simulink model "SequenceSeparation"  (R2018a)
settings: Solver=ode5  StartTime=0.0  StopTime=1  FixedStep=Ts  RelTol=1e-3
values from neighbouring files (symbols this model uses):
  Cdc = 2 * Sn * H / Vdc^2    (= 0.01875)    [SequenceSeparation_script.m]
  Cf = 1 / (wn * Xf)    (= 0.000159154943092)    [SequenceSeparation_script.m]
  Fn = 50    [SequenceSeparation_script.m]
  Kp_current = Rr * (Ti_current - halfTs)/(Tsum + halfTs)    [SequenceSeparation_script.m]
  Lr = Vdc / (0.8 * 2^0.5 * ( Sn / 3^0.5 / Vrms) * Fsw)    (= 0.00075)    [SequenceSeparation_script.m]
  Rf = 1 / ( 3 * 2 * pi * fres * Cf)    [SequenceSeparation_script.m]
  Rr = 0.005    [SequenceSeparation_script.m]
  Rt = 0.005    [SequenceSeparation_script.m]
  Sn = 1.5    [SequenceSeparation_script.m]
  Ts = 1e-6    (= 1e-06)    [SequenceSeparation_script.m]
  Ts_cont = 1/10000    (= 0.0001)    [SequenceSeparation_script.m]
  Ts_pwm = 1/200000    (= 5e-06)    [SequenceSeparation_script.m]
  Vdc = 2    [SequenceSeparation_script.m]
  Vrms = (3/2)^0.5    (= 1.22474487139)    [SequenceSeparation_script.m]
  Xr = Lr * wn    (= 0.235619449019)    [SequenceSeparation_script.m]
  Xt = 0.08    [SequenceSeparation_script.m]
undefined symbols (not defined in the file or in its folder): D1, Delta
libraries: powerlib x30, pwrsysVICtrl_202301 x6, pwrsysVSrc_202301 x2, pwrsysBasic_202301 x2, powerlib_meascontrol x1, pwrsysTransf_202301 x1
settings Model: Creator=daniemot  LastModifiedBy=daniemot

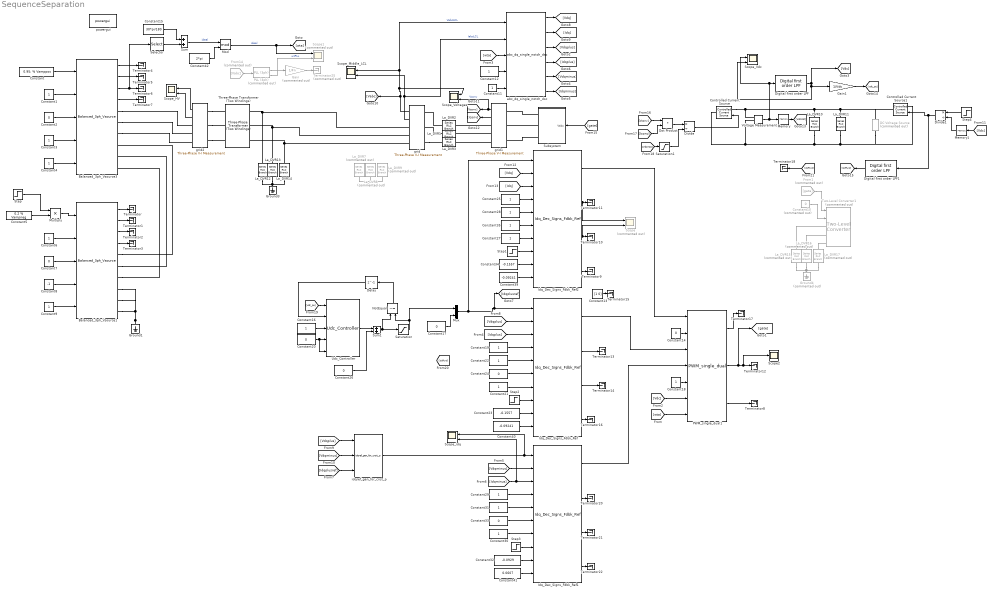
== system SequenceSeparation ==
  Balanced_3ph_Vsource1 : pwrsysVSrc_202301/Balanced_3ph_Vsource  BaseAmp=1  fn=50  AmpIni=1  SeqIni=1  AngIni=0  FIni=50  HarmIni=1
  Balanced_3ph_Vsource3 : pwrsysVSrc_202301/Balanced_3ph_Vsource  BaseAmp=1  fn=50  AmpIni=1  SeqIni=1  AngIni=0  FIni=50  HarmIni=1
  Constant : Constant  Value=0.95; % Vamppos
  Constant{1,3..4,6,9,11..12,16,18..19,21..22,25,27..31,35} (19 alike) : Constant
  Constant10 : Constant  Commented=on  Value=0
  Constant13 : Constant  Value=[1 0]
  Constant{2,7,14,17,20,24,26,33} (8 alike) : Constant  Value=0
  Constant15 : Constant  Value=30*pi/180
  Constant23 : Constant  Value=-0.1557
  Constant32 : Constant  Value=-0.0929
  Constant34 : Constant  Value=-0.1557
  Constant39 : Constant  Value=-0.09241
  Constant40 : Constant  Value=-0.09241
  Constant41 : Constant  Value=0.0607
  Constant42 : Constant  Value=2*pi
  Constant5 : Constant  Value=0.2 % Vampneg
  Constant8 : Constant  Value=-1
  Controlled Current Source : powerlib/Electrical Sources/Controlled Current Source  Initialize=on  Source_Type=AC  Amplitude=0  Phase=0  Frequency=0  Measurements=None
  Controlled Current Source1 : powerlib/Electrical Sources/Controlled Current Source  Initialize=on  Source_Type=AC  Amplitude=0  Phase=0  Frequency=0  Measurements=None
  DC Voltage Source : powerlib/Electrical Sources/DC Voltage Source  Commented=on  Amplitude=Vdc  Measurements=None
  Delay : Delay  DelayLength=1  SampleTime=Ts_cont
  Digital first order LPF : pwrsysBasic_202301/Digital first order LPF  Ts=Ts_cont  fcutout=fres
  Digital first order LPF1 : pwrsysBasic_202301/Digital first order LPF  Ts=Ts_cont  fcutout=fres
  Divide : Product  Inputs=*/
  Divide1 : Product  Inputs=*/
  Dot Product : DotProduct  InputSameDT=on  OutDataTypeStr=Inherit: Inherit via internal rule
  From1 : From  Commented=on  GotoTag=gate
  From14 : From  Commented=on  GotoTag=Vabc
  Gain : Gain  Commented=on  Gain=1/Fn
  Gain1 : Gain  Gain=1/Vdc
  Ground1 : powerlib/Elements/Ground  LConnTagsString=a
  Ground3 : powerlib/Elements/Ground  LConnTagsString=a
  Ground4 : powerlib/Elements/Ground  Commented=on  LConnTagsString=a
  Idq_Dec_Signs_Fdbk_Ref : pwrsysVICtrl_202301/Idq_Dec_Signs_Fdbk_Ref  Ts=Ts_cont  fn=Fn  Kp=Kp_current  Ti=Ti_current  L=Xr  PI_max=1.5  PI_min=-1.5  TrafoPhaseComp=0
  Idq_Dec_Signs_Fdbk_Ref1 : pwrsysVICtrl_202301/Idq_Dec_Signs_Fdbk_Ref  Ts=Ts_cont  fn=Fn  Kp=Kp_current  Ti=Ti_current  L=Xr  PI_max=1.5  PI_min=-1.5  TrafoPhaseComp=0
  Idq_Dec_Signs_Fdbk_Ref2 : pwrsysVICtrl_202301/Idq_Dec_Signs_Fdbk_Ref  Ts=Ts_cont  fn=Fn  Kp=Kp_current  Ti=Ti_current  L=Xr  PI_max=1.5  PI_min=-1.5  TrafoPhaseComp=0
  La_DVR1 : powerlib/Elements/Series RLC Branch  LConnTagsString=__new0  RConnTagsString=__new0  BranchType=RL  Resistance=Rr  Inductance=Lr  SetiL0=off  InitialCurrent=0  Capacitance=1.0  Setx0=off  InitialVoltage=0  Measurements=None
  La_DVR10 : powerlib/Elements/Series RLC Branch  LConnTagsString=__new0  RConnTagsString=__new0  BranchType=R  Resistance=100000  Inductance=0.3/(2*pi*50)  SetiL0=off  InitialCurrent=0  Capacitance=Cf  Setx0=off  InitialVoltage=0  Measurements=None
  La_DVR11 : powerlib/Elements/Series RLC Branch  LConnTagsString=__new0  RConnTagsString=__new0  BranchType=C  Resistance=100000  Inductance=0.3/(2*pi*50)  SetiL0=off  InitialCurrent=0  Capacitance=Cdc  Setx0=on  InitialVoltage=Vdc  Measurements=None
  La_DVR12 : powerlib/Elements/Series RLC Branch  LConnTagsString=__new0  RConnTagsString=__new0  BranchType=R  Resistance=1e6  Inductance=0.3/(2*pi*50)  SetiL0=off  InitialCurrent=0  Capacitance=1.0  Setx0=off  InitialVoltage=0  Measurements=None
  La_DVR13 : powerlib/Elements/Series RLC Branch  LConnTagsString=__new0  RConnTagsString=__new0  BranchType=R  Resistance=1e6  Inductance=0.3/(2*pi*50)  SetiL0=off  InitialCurrent=0  Capacitance=1.0  Setx0=off  InitialVoltage=0  Measurements=None
  La_DVR14 : powerlib/Elements/Series RLC Branch  LConnTagsString=__new0  RConnTagsString=__new0  BranchType=R  Resistance=1e6  Inductance=0.3/(2*pi*50)  SetiL0=off  InitialCurrent=0  Capacitance=1.0  Setx0=off  InitialVoltage=0  Measurements=None
  La_DVR15 : powerlib/Elements/Series RLC Branch  Commented=on  LConnTagsString=__new0  RConnTagsString=__new0  BranchType=R  Resistance=1e6  Inductance=0.3/(2*pi*50)  SetiL0=off  InitialCurrent=0  Capacitance=1.0  Setx0=off  InitialVoltage=0  Measurements=None
  La_DVR16 : powerlib/Elements/Series RLC Branch  Commented=on  LConnTagsString=__new0  RConnTagsString=__new0  BranchType=R  Resistance=1e6  Inductance=0.3/(2*pi*50)  SetiL0=off  InitialCurrent=0  Capacitance=1.0  Setx0=off  InitialVoltage=0  Measurements=None
  La_DVR17 : powerlib/Elements/Series RLC Branch  Commented=on  LConnTagsString=__new0  RConnTagsString=__new0  BranchType=R  Resistance=1e6  Inductance=0.3/(2*pi*50)  SetiL0=off  InitialCurrent=0  Capacitance=1.0  Setx0=off  InitialVoltage=0  Measurements=None
  La_DVR2 : powerlib/Elements/Series RLC Branch  LConnTagsString=__new0  RConnTagsString=__new0  BranchType=RL  Resistance=Rr  Inductance=Lr  SetiL0=off  InitialCurrent=0  Capacitance=1.0  Setx0=off  InitialVoltage=0  Measurements=None
  La_DVR3 : powerlib/Elements/Series RLC Branch  LConnTagsString=__new0  RConnTagsString=__new0  BranchType=RL  Resistance=Rr  Inductance=Lr  SetiL0=off  InitialCurrent=0  Capacitance=1.0  Setx0=off  InitialVoltage=0  Measurements=None
  La_DVR7 : powerlib/Elements/Series RLC Branch  Commented=on  LConnTagsString=__new0  RConnTagsString=__new0  BranchType=RC  Resistance=Rf  Inductance=0.3/(2*pi*50)  SetiL0=off  InitialCurrent=0  Capacitance=Cf  Setx0=off  InitialVoltage=0  Measurements=None
  La_DVR8 : powerlib/Elements/Series RLC Branch  Commented=on  LConnTagsString=__new0  RConnTagsString=__new0  BranchType=RC  Resistance=Rf  Inductance=0.3/(2*pi*50)  SetiL0=off  InitialCurrent=0  Capacitance=Cf  Setx0=off  InitialVoltage=0  Measurements=None
  La_DVR9 : powerlib/Elements/Series RLC Branch  Commented=on  LConnTagsString=__new0  RConnTagsString=__new0  BranchType=RC  Resistance=Rf  Inductance=0.3/(2*pi*50)  SetiL0=off  InitialCurrent=0  Capacitance=Cf  Setx0=off  InitialVoltage=0  Measurements=None
  Memory : Memory
  Memory1 : Memory  InitialCondition=1
  Mod : Math  Operator=mod  SaturateOnIntegerOverflow=on
  Multiply : Product
  Mux : Mux  Inputs=2
  NotEqual : RelationalOperator  Operator=~=  OutDataTypeStr=boolean  RndMeth=Simplest
  PLL (3ph) : powerlib_meascontrol/PLL/PLL (3ph)  Commented=on  Fmin=0.8*Fn  Par_Init=[0, Fn]  ParK=[180, 3200, 1]  TcD=1e-4  MaxRateChangeFreq=12  FilterCutOffFreq=25  Ts=Ts_cont  AGC=on
  PWM_single_dual1 : pwrsysVICtrl_202301/PWM_single_dual  fsw=Fsw  Ts=Ts_pwm  Uabp=Vampline  PWM_Ini_Phase=90
  Saturation : Saturate  UpperLimit=1.5  LowerLimit=-1.5
  Saturation1 : Saturate  UpperLimit=5  LowerLimit=0.25
  Scope : Scope  Commented=on  NumInputPorts=2
  Scope1 : Scope  Commented=on  NumInputPorts=2
  Scope2 : Scope
  Scope_HV : Scope  NumInputPorts=2
  Scope_Middle_LCL : Scope  NumInputPorts=2
  "Scope_Vdc " : Scope  NumInputPorts=2
  Scope_Voltages : Scope  NumInputPorts=2
  Scope_idq : Scope  NumInputPorts=2
  Selector : Selector  InputPortWidth=3  IndexOptions=Index vector (dialog)  Indices=[1]  OutputSizes=1
  Step : Step  Time=0.5  SampleTime=0
  Step1 : Step  Time=0.0002  After=0  SampleTime=0
  Step2 : Step  Time=0.0002  After=0  SampleTime=0
  Step3 : Step  Time=0.0002  After=0  SampleTime=0
  Step4 : Step  Time=0.25  After=0.25  SampleTime=0
  Subsystem : Subsystem
  Sum : Sum
  Sum1 : Sum
  Terminator{,1..18,20..22} (22 alike) : Terminator
  Terminator25 : Terminator  Commented=on
  Three-Phase Transformer (Two Windings) : powerlib/Elements/Three-Phase Transformer (Two Windings)  Winding1Connection=Delta (D1)  Winding2Connection=Y  CoreType=Three single-phase transformers  SetSaturation=off  Hysteresis=off  DataFile='hysteresis'  SetInitialFlux=off  Measurements=None  UNITS=pu  NominalPower=[ Sn , Fn ]  Winding1=[ Vrms , Rt , Xt ]  Winding2=[ Vrms , Rt , Xt ]  Rm=500  Lm=500  L0=0.5  Saturation=[ 0,0 ; 0.0024,1.2 ; 1.0,1.52 ]  InitialFluxes=[ 0.8 , -0.8 , 0.7 ]  MoreParameters=off  BreakLoop=off  DataType=off  TransfoNumber=1
  Two-Level Converter1 : powerlib/Power Electronics/Two-Level Converter  Commented=on  ModelType=Average model (Uref-controlled)  Ron=0.00001  Rs=1e6  Cs=inf  Vforward=[0,0]  Ron_Diode=0.001e-3  Rs_Diode=1e6  Cs_Diode=inf  Vf_Diode=1e-6  Rs_CurrentSource=inf
      settings: SourceProductName=Simscape Power Systems  SourceProductBaseCode=PS
  Udc_Controller : pwrsysVICtrl_202301/Udc_Controller  Ts=Ts_cont  Kp=5  Ti=0.025  PI_max=1.5  PI_min=-1.5
  Voltage Measurement : powerlib/Measurements/Voltage Measurement  PhasorSimulation=off  OutputType=Complex  PSBequivalent=0
  abc_dq_single_notch_dsc : pwrsysTransf_202301/abc_dq_single_notch_dsc  Ts=Ts_cont  fn=2*Fn  zeta=0.707
  grid : powerlib/Measurements/Three-Phase V-I Measurement  VoltageMeasurement=phase-to-ground  SetLabelV=off  LabelV=vgrid  Vpu=off  VpuLL=off  CurrentMeasurement=yes  SetLabelI=off  LabelI=igrid  Ipu=off  Pbase=sn  Vbase=uab  OutputType=Complex  PhasorSimulation=off  PSBequivalent=0
  grid1 : powerlib/Measurements/Three-Phase V-I Measurement  VoltageMeasurement=phase-to-ground  SetLabelV=off  LabelV=vgrid  Vpu=off  VpuLL=off  CurrentMeasurement=yes  SetLabelI=off  LabelI=igrid  Ipu=off  Pbase=sn  Vbase=uab  OutputType=Complex  PhasorSimulation=off  PSBequivalent=0
  grid2 : powerlib/Measurements/Three-Phase V-I Measurement  VoltageMeasurement=phase-to-ground  SetLabelV=off  LabelV=vgrid  Vpu=off  VpuLL=off  CurrentMeasurement=yes  SetLabelI=off  LabelI=igrid  Ipu=off  Pbase=sn  Vbase=uab  OutputType=Complex  PhasorSimulation=off  PSBequivalent=0
  idqref_gen_for_cnst_p : pwrsysVICtrl_202301/idqref_gen_for_cnst_p  Ts_control=Ts_cont
  powergui : powerlib/powergui  Priority=1  SimulationMode=Discrete  SampleTime=Ts  frequency=60  Iterations=50  frequencyindice=0  Pbase=100e6  ErrMax=1e-4  UnitsV=kV  UnitsW=MW  buscounter=0  FunctionMessages=off  echomessages=off  EnableUseOfTLC=off  CurrentSourceSwitches=off  DisableSnubberDevices=off  DisableRonSwitches=off  DisableVfSwitches=off  DisplayEquations=off  SolverType=Tustin/Backward Euler (TBE)  Interpol=off  ExternalGateDelay=off  methode=off  Ts=100  x0status=blocks  SPID=off  SwTol=0  HookPort=off  RestoreLinks=warning  ResistiveCurrentMeasurement=off  Frange=[60:1:1600]  Ylog=on  Xlog=on  ShowGrid=on  save=off  variable=ZData  structure=0  ZoomFFT=off  StartTime=0.0  cycles=1  DisplayStyle=1  fundamental=60  FreqAxis=off  MaxFrequency=1000  frequencyindicesteady=1  RmsSteady=1  display=off
  wires:
  Constant/1 -> Balanced_3ph_Vsource3/1
  Constant1/1 -> Balanced_3ph_Vsource3/2
  Constant2/1 -> Balanced_3ph_Vsource3/3
  Constant3/1 -> Balanced_3ph_Vsource3/4
  Constant4/1 -> Balanced_3ph_Vsource3/5
  Constant8/1 -> Balanced_3ph_Vsource1/4
  Constant5/1 -> Multiply/2
  Constant9/1 -> Balanced_3ph_Vsource1/5
  Constant6/1 -> Balanced_3ph_Vsource1/2
  Constant7/1 -> Balanced_3ph_Vsource1/3
  Balanced_3ph_Vsource1/1 -> Terminator/1
  Balanced_3ph_Vsource1/2 -> Terminator1/1
  Balanced_3ph_Vsource1/3 -> Terminator2/1
  Balanced_3ph_Vsource1/4 -> Terminator3/1
  Balanced_3ph_Vsource3/1 -> Terminator4/1
  Balanced_3ph_Vsource3/4 -> Terminator7/1
  Balanced_3ph_Vsource3/2 -> Terminator5/1
  Balanced_3ph_Vsource3/3 -> Selector/1, Terminator6/1
  Selector/1 -> Sum/2
  Mod/1 -> Scope1/1, [wta]  "ideal"
  Constant15/1 -> Sum/1
  Saturation/1 -> Mux/1, NotEqual/2
  [wta] -> PWM_single_dual1/7
  Constant10/1 -> Two-Level Converter1/2
  From1/1 -> Two-Level Converter1/1
  PWM_single_dual1/2 -> [gate], Scope2/1, Terminator12/1
  Constant11/1 -> abc_dq_single_notch_dsc/5
  [wta] -> abc_dq_single_notch_dsc/3
  Constant12/1 -> abc_dq_single_notch_dsc/4
  [Vdc] -> PWM_single_dual1/6
  PWM_single_dual1/1 -> Terminator17/1
  PWM_single_dual1/3 -> Terminator8/1
  Constant14/1 -> PWM_single_dual1/2
  Constant18/1 -> PWM_single_dual1/5
  Constant19/1 -> Idq_Dec_Signs_Fdbk_Ref/4
  Constant21/1 -> Idq_Dec_Signs_Fdbk_Ref/7
  Constant22/1 -> Idq_Dec_Signs_Fdbk_Ref/5
  Constant24/1 -> Idq_Dec_Signs_Fdbk_Ref/6
  [Vdqplus] -> Idq_Dec_Signs_Fdbk_Ref/2
  Idq_Dec_Signs_Fdbk_Ref/2 -> Terminator13/1
  Idq_Dec_Signs_Fdbk_Ref/3 -> Terminator14/1
  Idq_Dec_Signs_Fdbk_Ref/4 -> Terminator16/1
  grid/1 -> [Vabc], Scope_Voltages/1, abc_dq_single_notch_dsc/1, Scope_Middle_LCL/1  "VabcLCL"
  grid/2 -> abc_dq_single_notch_dsc/2, Scope_Middle_LCL/2  "IabcLCL"
  grid1/1 -> [Vconv], Scope_Voltages/2  "Vconv"
  grid1/2 -> [Iconv]
  Multiply/1 -> Balanced_3ph_Vsource1/1
  Step/1 -> Multiply/1
  Constant29/1 -> Idq_Dec_Signs_Fdbk_Ref1/4
  [Vdqminus] -> Idq_Dec_Signs_Fdbk_Ref1/2
  Idq_Dec_Signs_Fdbk_Ref1/2 -> Terminator20/1
  [Idqminus] -> Scope_idq/2, Idq_Dec_Signs_Fdbk_Ref1/3
  Idq_Dec_Signs_Fdbk_Ref1/3 -> Terminator21/1
  Constant30/1 -> Idq_Dec_Signs_Fdbk_Ref1/7
  Idq_Dec_Signs_Fdbk_Ref1/4 -> Terminator22/1
  Constant33/1 -> Idq_Dec_Signs_Fdbk_Ref1/6
  Constant31/1 -> Idq_Dec_Signs_Fdbk_Ref1/5
  abc_dq_single_notch_dsc/3 -> [Vdqplus]
  abc_dq_single_notch_dsc/5 -> [Vdqminus]
  abc_dq_single_notch_dsc/6 -> [Idqminus]
  abc_dq_single_notch_dsc/4 -> [Idqplus]
  [Idqplusref] -> idqref_gen_for_cnst_p/3
  [Vdqplus] -> idqref_gen_for_cnst_p/1
  [Vdqminus] -> idqref_gen_for_cnst_p/2
  abc_dq_single_notch_dsc/1 -> [Vdq]
  abc_dq_single_notch_dsc/2 -> [Idq]
  Constant20/1 -> Udc_Controller/5, Udc_Controller/4
  Constant16/1 -> Udc_Controller/3
  Udc_Controller/1 -> Sum1/1
  Sum1/1 -> NotEqual/1, Saturation/1
  Constant26/1 -> Sum1/2
  Delay/1 -> Udc_Controller/2
  Digital first order LPF/1 -> Gain1/1, "Scope_Vdc "/2, [Vdc]
  Voltage Measurement/1 -> Memory/1, Digital first order LPF/1, "Scope_Vdc "/1
  [vdc_pu] -> Udc_Controller/1
  Constant25/1 -> Idq_Dec_Signs_Fdbk_Ref2/4
  Constant28/1 -> Idq_Dec_Signs_Fdbk_Ref2/5
  Constant35/1 -> Idq_Dec_Signs_Fdbk_Ref2/6
  Constant27/1 -> Idq_Dec_Signs_Fdbk_Ref2/7
  Step1/1 -> Idq_Dec_Signs_Fdbk_Ref2/8
  [Vdq] -> Idq_Dec_Signs_Fdbk_Ref2/2
  [Idq] -> Idq_Dec_Signs_Fdbk_Ref2/3
  Idq_Dec_Signs_Fdbk_Ref2/4 -> Terminator9/1
  Idq_Dec_Signs_Fdbk_Ref2/3 -> Scope/2, Terminator10/1
  Idq_Dec_Signs_Fdbk_Ref2/2 -> Scope/1, Terminator11/1
  Constant13/1 -> Terminator15/1
  Idq_Dec_Signs_Fdbk_Ref2/1 -> PWM_single_dual1/1
  idqref_gen_for_cnst_p/1 -> Scope_idq/1, Idq_Dec_Signs_Fdbk_Ref1/1
  grid2/1 -> Scope_HV/1
  grid2/2 -> Scope_HV/2
  Constant34/1 -> Idq_Dec_Signs_Fdbk_Ref2/9
  Constant39/1 -> Idq_Dec_Signs_Fdbk_Ref2/10
  Step2/1 -> Idq_Dec_Signs_Fdbk_Ref/8
  Constant40/1 -> Idq_Dec_Signs_Fdbk_Ref/10
  Constant23/1 -> Idq_Dec_Signs_Fdbk_Ref/9
  Constant32/1 -> Idq_Dec_Signs_Fdbk_Ref1/9
  Constant41/1 -> Idq_Dec_Signs_Fdbk_Ref1/10
  Step3/1 -> Idq_Dec_Signs_Fdbk_Ref1/8
  From14/1 -> PLL (3ph)/1
  PLL (3ph)/1 -> Gain/1
  Gain/1 -> Terminator25/1
  PLL (3ph)/2 -> Scope1/2  "wtPLL"
  Sum/1 -> Mod/1  "ideal"
  Constant42/1 -> Mod/2
  [Idqplus] -> Idq_Dec_Signs_Fdbk_Ref/3
  Idq_Dec_Signs_Fdbk_Ref/1 -> PWM_single_dual1/3
  Idq_Dec_Signs_Fdbk_Ref1/1 -> PWM_single_dual1/4
  [gate] -> Subsystem/1(Vabc)
  [Vconv] -> Dot Product/1
  [Iconv] -> Dot Product/2
  Memory/1 -> [Vdcinst]
  Dot Product/1 -> Divide/1
  [Vdcinst] -> Saturation1/1
  Saturation1/1 -> Divide/2
  Divide/1 -> Controlled Current Source/1
  NotEqual/1 -> Delay/1
  Gain1/1 -> [vdc_pu]
  Mux/1 -> Idq_Dec_Signs_Fdbk_Ref2/1, [Idqplusref], Idq_Dec_Signs_Fdbk_Ref/1
  Constant17/1 -> Mux/2
  Step4/1 -> Divide1/1
  Divide1/1 -> Digital first order LPF1/1, Controlled Current Source1/1
  [Vdc] -> Memory1/1
  Memory1/1 -> Divide1/2
  Digital first order LPF1/1 -> [idcffwrd]
  [idcffwrd] -> Terminator18/1
  connections:
  Ground1/LConn1 -- Balanced_3ph_Vsource1/RConn6 -- Balanced_3ph_Vsource1/RConn5 -- Balanced_3ph_Vsource1/RConn4
  Balanced_3ph_Vsource1/RConn3 -- Balanced_3ph_Vsource3/RConn6
  Balanced_3ph_Vsource1/RConn2 -- Balanced_3ph_Vsource3/RConn5
  Balanced_3ph_Vsource1/RConn1 -- Balanced_3ph_Vsource3/RConn4
  Balanced_3ph_Vsource3/RConn1 -- grid2/RConn1
  Balanced_3ph_Vsource3/RConn2 -- grid2/RConn2
  Balanced_3ph_Vsource3/RConn3 -- grid2/RConn3
  Voltage Measurement/LConn1 -- DC Voltage Source/RConn1 -- Controlled Current Source1/RConn1 -- La_DVR11/LConn1 -- La_DVR10/LConn1 -- Controlled Current Source/LConn1
  Voltage Measurement/LConn2 -- Controlled Current Source/RConn1 -- DC Voltage Source/LConn1 -- Controlled Current Source1/LConn1 -- La_DVR11/RConn1 -- La_DVR10/RConn1
  La_DVR9/LConn1 -- La_DVR7/LConn1 -- La_DVR8/LConn1
  grid1/RConn1 -- La_DVR2/LConn1
  grid1/RConn2 -- La_DVR1/LConn1
  grid1/RConn3 -- La_DVR3/LConn1
  grid/LConn3 -- La_DVR3/RConn1
  La_DVR1/RConn1 -- grid/LConn2
  La_DVR2/RConn1 -- grid/LConn1
  grid2/LConn1 -- Three-Phase Transformer (Two Windings)/LConn1
  grid2/LConn2 -- Three-Phase Transformer (Two Windings)/LConn2
  grid2/LConn3 -- Three-Phase Transformer (Two Windings)/LConn3
  La_DVR12/LConn1 -- La_DVR14/LConn1 -- La_DVR13/LConn1 -- Ground3/LConn1
  La_DVR14/RConn1 -- grid/RConn3 -- Three-Phase Transformer (Two Windings)/RConn3
  La_DVR13/RConn1 -- grid/RConn2 -- Three-Phase Transformer (Two Windings)/RConn2
  La_DVR12/RConn1 -- grid/RConn1 -- Three-Phase Transformer (Two Windings)/RConn1
  La_DVR15/LConn1 -- La_DVR17/LConn1 -- La_DVR16/LConn1 -- Ground4/LConn1
  Two-Level Converter1/LConn1 -- La_DVR15/RConn1
  Two-Level Converter1/LConn2 -- La_DVR16/RConn1
  Two-Level Converter1/LConn3 -- La_DVR17/RConn1
  Subsystem/RConn1 -- grid1/LConn1
  Subsystem/RConn2 -- grid1/LConn2
  Subsystem/RConn3 -- grid1/LConn3

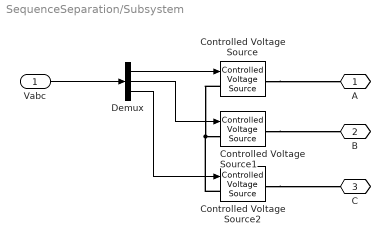
== system SequenceSeparation/Subsystem ==
  Vabc : Inport
  Controlled Voltage Source : powerlib/Electrical Sources/Controlled Voltage Source  Initialize=off  Source_Type=DC  Amplitude=0  Phase=0  Frequency=0  Measurements=None
  Controlled Voltage Source1 : powerlib/Electrical Sources/Controlled Voltage Source  Initialize=off  Source_Type=DC  Amplitude=0  Phase=0  Frequency=0  Measurements=None
  Controlled Voltage Source2 : powerlib/Electrical Sources/Controlled Voltage Source  Initialize=off  Source_Type=DC  Amplitude=0  Phase=0  Frequency=0  Measurements=None
  Demux : Demux  Outputs=3
  A : PMIOPort  Side=Right
  B : PMIOPort  Port=2  Side=Right
  C : PMIOPort  Port=3  Side=Right
  wires:
  Vabc/1 -> Demux/1
  Demux/2 -> Controlled Voltage Source1/1
  Demux/1 -> Controlled Voltage Source/1
  Demux/3 -> Controlled Voltage Source2/1
  connections:
  Controlled Voltage Source/LConn1 -- Controlled Voltage Source2/LConn1 -- Controlled Voltage Source1/LConn1
  Controlled Voltage Source1/RConn1 -- B/RConn1
  Controlled Voltage Source2/RConn1 -- C/RConn1
  Controlled Voltage Source/RConn1 -- A/RConn1
